simulink model "IMC"  (Simulink 7.6)
settings: Solver=ode45  StartTime=0.0  StopTime=10.0  RelTol=1e-3
values from neighbouring files (symbols this model uses):
  clight = 2.99e8    (= 299000000)    [Generate_IMC_Simulink.m]
  imcl =     [IMC_Filters.mat]
  lambda = 1.064e-6    (= 1.064e-06)    [Generate_IMC_Simulink.m]
  mc2m1l = -1/12*mc2m1l    [ArbLoop_IMC_Simple.m]    (also in IMC_Filters.mat = )
  mc2m2l =     [IMC_Filters.mat]
  mc2m3l = 2.25*mc2m3l    [ArbLoop_IMC_Simple.m]    (also in IMC_Filters.mat = )
  sus =     [sus.mat]
undefined symbols (not defined in the file or in its folder): imc
libraries: cstblocks x42, simulink x16
settings Model: Creator=adammullavey  LastModifiedBy=Chris Mueller
settings DebuggingCC: FcnCallInpInsideContextMsg=Enable All

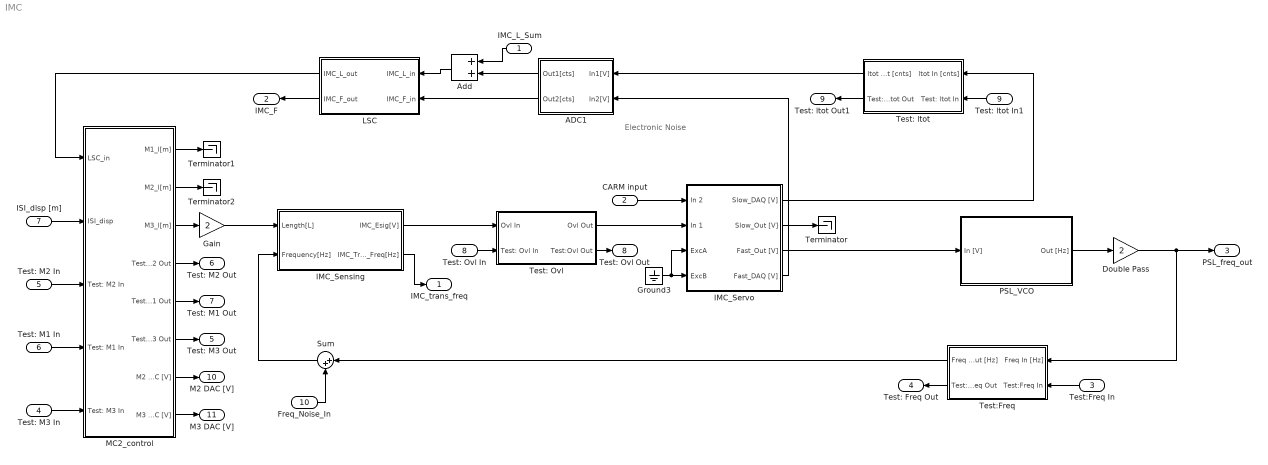
== system IMC ==
  note: Electronic Noise
  IMC_L_Sum : Inport
  CARM input : Inport  Port=2
  Test:Freq In : Inport  Port=3
  Test: M3 In : Inport  Port=4
  Test: M2 In : Inport  Port=5
  Test: M1 In : Inport  Port=6
  ISI_disp [m] : Inport  Port=7
  Test: Ovl In : Inport  Port=8
  Test: ltot In1 : Inport  Port=9
  Freq_Noise_In : Inport  Port=10
  ADC1 : Subsystem
  Add : Sum
  Double Pass : Gain  Gain=2
  Gain : Gain  Gain=2
  Ground3 : Ground
  IMC_Sensing : Subsystem
  IMC_Servo : Subsystem
  LSC : Subsystem
  MC2_control : Subsystem
  PSL_VCO : Subsystem
  Sum : Sum  Inputs=|++
  Terminator : Terminator
  Terminator1 : Terminator
  Terminator2 : Terminator
  Test: Ovl : Subsystem
  Test: ltot : Subsystem
  Test:Freq : Subsystem
  IMC_trans_freq : Outport
  IMC_F : Outport  Port=2
  PSL_freq_out : Outport  Port=3
  Test: Freq Out : Outport  Port=4
  Test: M3 Out : Outport  Port=5
  Test: M2 Out : Outport  Port=6
  Test: M1 Out : Outport  Port=7
  Test: Ovl Out : Outport  Port=8
  Test: ltot Out1 : Outport  Port=9
  M2 DAC [V] : Outport  Port=10
  M3 DAC [V] : Outport  Port=11
  wires:
  Ground3/1 -> IMC_Servo/4(ExcB), IMC_Servo/3(ExcA)
  IMC_Sensing/2(IMC_Trans_Freq[Hz]) -> IMC_trans_freq/1
  IMC_Servo/4(Fast_DAQ [V]) -> ADC1/2(In2[V])
  ADC1/2(Out2[cts]) -> LSC/2(IMC_F_in)
  IMC_Servo/2(Slow_Out [V]) -> Terminator/1
  MC2_control/1(M1_l[m]) -> Terminator1/1
  LSC/2(IMC_F_out) -> IMC_F/1
  PSL_VCO/1(Out [Hz]) -> Double Pass/1
  Double Pass/1 -> PSL_freq_out/1, Test:Freq/1(Freq In [Hz])
  CARM input/1 -> IMC_Servo/1(In 2)
  Gain/1 -> IMC_Sensing/1(Length[L])
  IMC_Servo/3(Fast_Out [V]) -> PSL_VCO/1(In [V])
  Test:Freq In/1 -> Test:Freq/2(Test:Freq In)
  Test:Freq/2(Test:Freq Out) -> Test: Freq Out/1
  LSC/1(IMC_L_out) -> MC2_control/1(LSC_in)
  MC2_control/3(M3_l[m]) -> Gain/1
  MC2_control/2(M2_l[m]) -> Terminator2/1
  Test: M2 In/1 -> MC2_control/3(Test: M2 In)
  MC2_control/4(Test: M2 Out) -> Test: M2 Out/1
  MC2_control/5(Test: M1 Out) -> Test: M1 Out/1
  Test: M1 In/1 -> MC2_control/4(Test: M1 In)
  Test: M3 In/1 -> MC2_control/5(Test: M3 In)
  MC2_control/6(Test: M3 Out) -> Test: M3 Out/1
  Add/1 -> LSC/1(IMC_L_in)
  IMC_L_Sum/1 -> Add/1
  ADC1/1(Out1[cts]) -> Add/2
  ISI_disp [m]/1 -> MC2_control/2(ISI_disp)
  Test: Ovl/2(Test:Ovl Out) -> Test: Ovl Out/1
  Test: Ovl In/1 -> Test: Ovl/2(Test: Ovl In)
  IMC_Sensing/1(IMC_Esig[V]) -> Test: Ovl/1(Ovl In)
  Test: Ovl/1(Ovl Out) -> IMC_Servo/2(In 1)
  Test: ltot/2(Test: ltot Out) -> Test: ltot Out1/1
  Test: ltot In1/1 -> Test: ltot/2(Test: ltot In)
  IMC_Servo/1(Slow_DAQ [V]) -> Test: ltot/1(ltot In [cnts])
  MC2_control/7(M2 DAC [V]) -> M2 DAC [V]/1
  MC2_control/8(M3 DAC [V]) -> M3 DAC [V]/1
  Test: ltot/1(ltot Out [cnts]) -> ADC1/1(In1[V])
  Test:Freq/1(Freq Out [Hz]) -> Sum/1
  Sum/1 -> IMC_Sensing/2(Frequency[Hz])
  Freq_Noise_In/1 -> Sum/2

== system IMC/ADC1 ==
  In1[V] : Inport
  In2[V] : Inport  Port=2
  Gain : Gain  Gain=(2^16)/40
  Gain1 : Gain  Gain=(2^16)/40
  Out1[cts] : Outport
  Out2[cts] : Outport  Port=2
  wires:
  Gain/1 -> Out1[cts]/1
  In1[V]/1 -> Gain/1
  Gain1/1 -> Out2[cts]/1
  In2[V]/1 -> Gain1/1

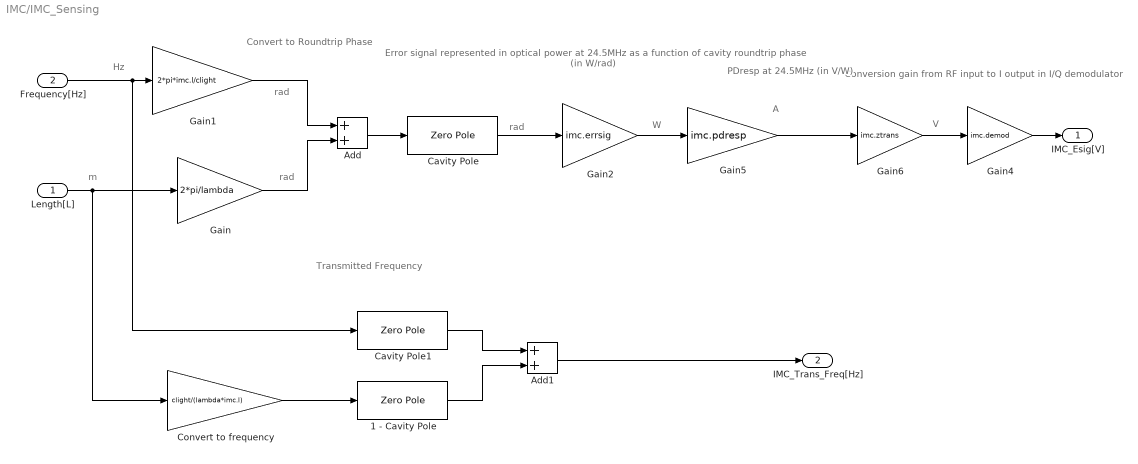
== system IMC/IMC_Sensing ==
  note: Hz
  note: rad
  note: rad
  note: rad
  note: m
  note: V
  note: W
  note: Conversion gain from
      | RF input to I output
      | in I/Q demodulator
  note: Convert to
      | Roundtrip Phase
  note: Error signal represented in
      | optical power at 24.5MHz
      | as a function of cavity
      | roundtrip phase (in W/rad)
  note: Transmitted Frequency
  note: PDresp at 24.5MHz
      |  (in V/W)
  note: A
  Length[L] : Inport
  Frequency[Hz] : Inport  Port=2
  1 - Cavity Pole : ZeroPole  Zeros=[0]  Poles=[-imc.p]  Gain=1
  Add : Sum
  Add1 : Sum
  Cavity Pole : ZeroPole  Zeros=[]  Poles=[-imc.p]  Gain=[imc.p]
  Cavity Pole1 : ZeroPole  Zeros=[]  Poles=[-imc.p]  Gain=[imc.p]
  Convert to frequency : Gain  Gain=clight/(lambda*imc.l)
  Gain : Gain  Gain=2*pi/lambda
  Gain1 : Gain  Gain=2*pi*imc.l/clight
  Gain2 : Gain  Gain=imc.errsig
  Gain4 : Gain  Gain=imc.demod
  Gain5 : Gain  Gain=imc.pdresp
  Gain6 : Gain  Gain=imc.ztrans
  IMC_Esig[V] : Outport
  IMC_Trans_Freq[Hz] : Outport  Port=2
  wires:
  Length[L]/1 -> Convert to frequency/1, Gain/1
  Frequency[Hz]/1 -> Gain1/1, Cavity Pole1/1
  Gain1/1 -> Add/1
  Gain/1 -> Add/2
  Add/1 -> Cavity Pole/1
  Cavity Pole/1 -> Gain2/1
  Add1/1 -> IMC_Trans_Freq[Hz]/1
  Gain4/1 -> IMC_Esig[V]/1
  Gain2/1 -> Gain5/1
  Gain6/1 -> Gain4/1
  Gain5/1 -> Gain6/1
  Cavity Pole1/1 -> Add1/1
  Convert to frequency/1 -> 1 - Cavity Pole/1
  1 - Cavity Pole/1 -> Add1/2

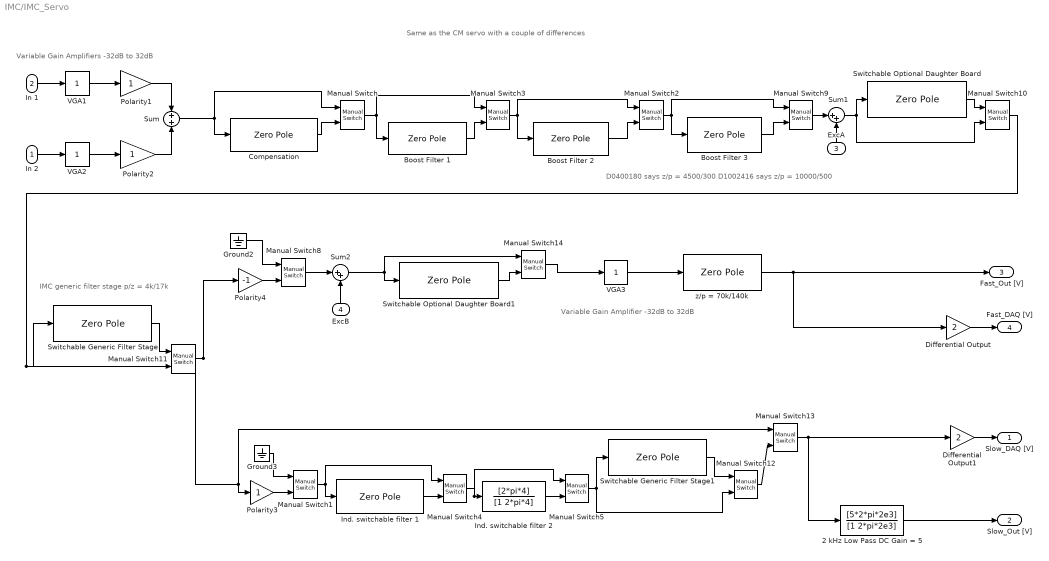
== system IMC/IMC_Servo ==
  note: IMC generic filter stage
      | p/z = 4k/17k
  note: Same as the CM servo with a couple of differences
  note: D0400180 says z/p = 4500/300
      | D1002416 says z/p = 10000/500
  note: Variable Gain Amplifier
      | -32dB to 32dB
  note: Variable Gain Amplifiers
      | -32dB to 32dB
  In 2 : Inport
  In 1 : Inport  Port=2
  ExcA : Inport  Port=3
  ExcB : Inport  Port=4
  2 kHz Low Pass DC Gain = 5 : TransferFcn  Numerator=[5*2*pi*2e3]  Denominator=[1 2*pi*2e3]
  Boost Filter 1 : ZeroPole  Zeros=-2*pi*[20e3]  Poles=-2*pi*[1e3]
  Boost Filter 2 : ZeroPole  Zeros=-2*pi*[20e3]  Poles=-2*pi*[1e3]
  Boost Filter 3 : ZeroPole  Zeros=-2*pi*[10e3]  Poles=-2*pi*[500]
  Compensation : ZeroPole  Zeros=-2*pi*[4e3]  Poles=-2*pi*[40]
  Differential Output : Gain  Gain=2
  Differential Output1 : Gain  Gain=2
  Ground2 : Ground
  Ground3 : Ground
  Ind. switchable filter 1 : ZeroPole  Zeros=-2*pi*[400]  Poles=-2*pi*[4]  Gain=[1/100]
  Ind. switchable filter 2 : TransferFcn  Numerator=[2*pi*4]  Denominator=[1 2*pi*4]
  Manual Switch{,1,3..4,8,10..12} (8 alike) : simulink/Signal Routing/Manual Switch  SystemSampleTime=-1  sw=0  action=0  varsize=off
  Manual Switch{2,5,9,13..14} (5 alike) : simulink/Signal Routing/Manual Switch  SystemSampleTime=-1  sw=1  action=0  varsize=off
  Polarity1 : Gain
  Polarity2 : Gain
  Polarity3 : Gain
  Polarity4 : Gain  Gain=-1
  Sum : Sum  Inputs=+|+
  Sum1 : Sum  Inputs=|++
  Sum2 : Sum  Inputs=|++
  Switchable Generic Filter Stage : ZeroPole  Zeros=-2*pi*[17e3]  Poles=-2*pi*[4e3]  Gain=[4/17]
  Switchable Generic Filter Stage1 : ZeroPole  Zeros=-2*pi*[500]  Poles=-2*pi*[1e4]  Gain=[1e4/500]
  Switchable Optional Daughter Board : ZeroPole  Zeros=-2*pi*[500]  Poles=-2*pi*[1e4]  Gain=[1e4/500]
  Switchable Optional Daughter Board1 : ZeroPole  Zeros=-2*pi*[500]  Poles=-2*pi*[1e4]  Gain=[1e4/500]
  VGA1 : simulink/Math Operations/Slider Gain  SystemSampleTime=-1  low=0.025  gain=1  high=40
  VGA2 : simulink/Math Operations/Slider Gain  SystemSampleTime=-1  low=0.025  gain=1  high=40
  VGA3 : simulink/Math Operations/Slider Gain  SystemSampleTime=-1  low=0.025  gain=1  high=40
  z/p = 70k/140k : ZeroPole  Zeros=-2*pi*[70000]  Poles=-2*pi*[140000]  Gain=2
  Slow_DAQ [V] : Outport
  Slow_Out [V] : Outport  Port=2
  Fast_Out [V] : Outport  Port=3
  Fast_DAQ [V] : Outport  Port=4
  wires:
  Polarity1/1 -> Sum/1
  VGA1/1 -> Polarity1/1
  In 1/1 -> VGA1/1
  VGA3/1 -> z/p = 70k/140k/1
  VGA2/1 -> Polarity2/1
  In 2/1 -> VGA2/1
  Switchable Generic Filter Stage1/1 -> Manual Switch12/1
  Ground3/1 -> Manual Switch1/1
  Ground2/1 -> Manual Switch8/1
  Switchable Optional Daughter Board1/1 -> Manual Switch14/2
  Compensation/1 -> Manual Switch/2
  Manual Switch/1 -> Manual Switch3/1, Boost Filter 1/1
  Boost Filter 1/1 -> Manual Switch3/2
  Manual Switch3/1 -> Manual Switch2/1, Boost Filter 2/1
  Boost Filter 2/1 -> Manual Switch2/2
  Switchable Optional Daughter Board/1 -> Manual Switch10/1
  Manual Switch1/1 -> Manual Switch4/1, Ind. switchable filter 1/1
  Manual Switch4/1 -> Manual Switch5/1, Ind. switchable filter 2/1
  Manual Switch5/1 -> Switchable Generic Filter Stage1/1, Manual Switch12/2
  Ind. switchable filter 2/1 -> Manual Switch5/2
  Sum/1 -> Manual Switch/1, Compensation/1
  ExcB/1 -> Sum2/2
  Manual Switch8/1 -> Sum2/1
  z/p = 70k/140k/1 -> Fast_Out [V]/1, Differential Output/1
  Polarity2/1 -> Sum/2
  ExcA/1 -> Sum1/2
  Boost Filter 3/1 -> Manual Switch9/2
  Manual Switch9/1 -> Sum1/1
  Manual Switch2/1 -> Manual Switch9/1, Boost Filter 3/1
  Ind. switchable filter 1/1 -> Manual Switch4/2
  Sum1/1 -> Switchable Optional Daughter Board/1, Manual Switch10/2
  Manual Switch10/1 -> Switchable Generic Filter Stage/1, Manual Switch11/2
  Switchable Generic Filter Stage/1 -> Manual Switch11/1
  Manual Switch11/1 -> Manual Switch13/1, Polarity3/1, Polarity4/1
  Manual Switch12/1 -> Manual Switch13/2
  Sum2/1 -> Switchable Optional Daughter Board1/1, Manual Switch14/1
  Manual Switch14/1 -> VGA3/1
  Polarity4/1 -> Manual Switch8/2
  Polarity3/1 -> Manual Switch1/2
  Manual Switch13/1 -> 2 kHz Low Pass DC Gain = 5/1, Differential Output1/1
  Differential Output/1 -> Fast_DAQ [V]/1
  2 kHz Low Pass DC Gain = 5/1 -> Slow_Out [V]/1
  Differential Output1/1 -> Slow_DAQ [V]/1

== system IMC/LSC ==
  note: Copied from foton
  IMC_L_in : Inport
  IMC_F_in : Inport  Port=2
  IMC-L Filter Bank : Subsystem
  InvGenFilt : ZeroPole  Zeros=-2*pi*[100 100]  Poles=-2*pi*[10 10]  Gain=[0.01/2]
  VCO  filter [cts/cts]:  pole:1.6 Hz; zero:40 Hz : ZeroPole  Zeros=-2*pi*[40]  Poles=-2*pi*[1.6]  Gain=1.4906e6*(1.6/40)
  ctstoV : Gain  Gain=6.10016e-4
  IMC_L_out : Outport
  IMC_F_out : Outport  Port=2
  wires:
  IMC_L_in/1 -> IMC-L Filter Bank/1(In1)
  IMC-L Filter Bank/1(Out1) -> IMC_L_out/1
  IMC_F_in/1 -> InvGenFilt/1
  InvGenFilt/1 -> VCO  filter [cts/cts]:  pole:1.6 Hz; zero:40 Hz/1
  VCO  filter [cts/cts]:  pole:1.6 Hz; zero:40 Hz/1 -> ctstoV/1
  ctstoV/1 -> IMC_F_out/1

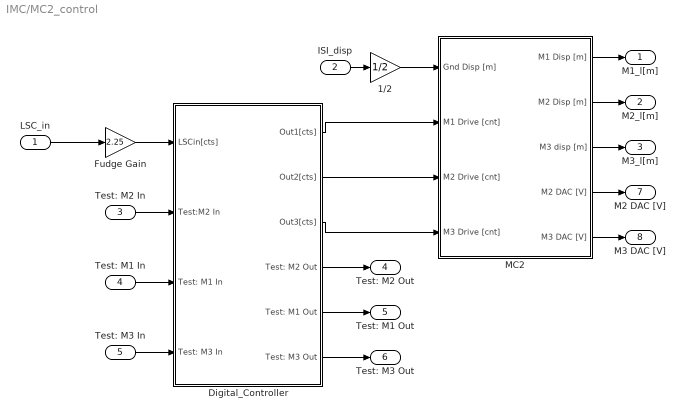
== system IMC/MC2_control ==
  LSC_in : Inport
  ISI_disp : Inport  Port=2
  Test: M2 In : Inport  Port=3
  Test: M1 In : Inport  Port=4
  Test: M3 In : Inport  Port=5
  1/2 : Gain  Gain=1/2
  Digital_Controller : Subsystem
  Fudge Gain : Gain  Gain=2.25
  MC2 : Subsystem
  M1_l[m] : Outport
  M2_l[m] : Outport  Port=2
  M3_l[m] : Outport  Port=3
  Test: M2 Out : Outport  Port=4
  Test: M1 Out : Outport  Port=5
  Test: M3 Out : Outport  Port=6
  M2 DAC [V] : Outport  Port=7
  M3 DAC [V] : Outport  Port=8
  wires:
  ISI_disp/1 -> 1/2/1
  MC2/2(M2 Disp [m]) -> M2_l[m]/1
  MC2/1(M1 Disp [m]) -> M1_l[m]/1
  MC2/3(M3 disp [m]) -> M3_l[m]/1
  Digital_Controller/1(Out1[cts]) -> MC2/2(M1 Drive [cnt])
  Digital_Controller/2(Out2[cts]) -> MC2/3(M2 Drive [cnt])
  Digital_Controller/3(Out3[cts]) -> MC2/4(M3 Drive [cnt])
  LSC_in/1 -> Fudge Gain/1
  Test: M2 In/1 -> Digital_Controller/2(Test:M2 In)
  Test: M1 In/1 -> Digital_Controller/3(Test: M1 In)
  Digital_Controller/4(Test: M2 Out) -> Test: M2 Out/1
  Digital_Controller/5(Test: M1 Out) -> Test: M1 Out/1
  Test: M3 In/1 -> Digital_Controller/4(Test: M3 In)
  Digital_Controller/6(Test: M3 Out) -> Test: M3 Out/1
  Fudge Gain/1 -> Digital_Controller/1(LSCin[cts])
  MC2/4(M2 DAC [V]) -> M2 DAC [V]/1
  MC2/5(M3 DAC [V]) -> M3 DAC [V]/1
  1/2/1 -> MC2/1(Gnd Disp [m])

== system IMC/PSL_VCO ==
  note: Output range of +/-1MHz (79-81MHz), Input range +/-20V, hence sensitivity 1MHz/20V. Just an approximation, really should be measured.
  note: Low Noise VCO - described in T0900451, schematics in D0900605-A
  note: P/Z = 275kHz/2750kHz
  note: 1MHz/20V
  note: llo alog 4090 - old VCO = 745300Hz/V
  note: valera says new vco = old vco/3
      | therefore new vco = 2.4843e5 Hz/V
  In [V] : Inport
  VCO  filter [V/V]:  pole:1.6 Hz; zero:40 Hz : ZeroPole  Zeros=-2*pi*[40]  Poles=-2*pi*[1.6]  Gain=(1.6/40)
  VCO TF req - 20 deg phase shift at 50 kHz : ZeroPole  Zeros=-2*pi*[2750e3]  Poles=-2*pi*[275e3]  Gain=(1/10)
  VCO gain [Hz/V] : Gain  Gain=2.4843e5  SaturateOnIntegerOverflow=on  OutDataTypeStr=Inherit: Same as input  ParamDataTypeStr=Inherit: Same as input
  Out [Hz] : Outport
  wires:
  In [V]/1 -> VCO  filter [V/V]:  pole:1.6 Hz; zero:40 Hz/1
  VCO gain [Hz/V]/1 -> Out [Hz]/1
  VCO  filter [V/V]:  pole:1.6 Hz; zero:40 Hz/1 -> VCO TF req - 20 deg phase shift at 50 kHz/1
  VCO TF req - 20 deg phase shift at 50 kHz/1 -> VCO gain [Hz/V]/1

== system IMC/Test: Ovl ==
  Ovl In : Inport
  Test: Ovl In : Inport  Port=2
  Add : Sum
  Constant : Constant  Value=imc.sw.ovl
  Ground : Ground
  Switch : Switch  Threshold=0.5
  Ovl Out : Outport
  Test:Ovl Out : Outport  Port=2
  wires:
  Ground/1 -> Switch/3
  Constant/1 -> Switch/2
  Ovl In/1 -> Switch/1, Test:Ovl Out/1
  Switch/1 -> Add/2
  Test: Ovl In/1 -> Add/1
  Add/1 -> Ovl Out/1

== system IMC/Test: ltot ==
  ltot In [cnts] : Inport
  Test: ltot In : Inport  Port=2
  Add : Sum
  Constant : Constant  Value=imc.sw.ltot
  Ground : Ground
  Switch : Switch  Threshold=0.5
  ltot Out [cnts] : Outport
  Test: ltot Out : Outport  Port=2
  wires:
  Add/1 -> ltot Out [cnts]/1
  Test: ltot In/1 -> Add/1
  Switch/1 -> Add/2
  ltot In [cnts]/1 -> Test: ltot Out/1, Switch/1
  Constant/1 -> Switch/2
  Ground/1 -> Switch/3

== system IMC/Test:Freq ==
  Freq In [Hz] : Inport
  Test:Freq In : Inport  Port=2
  Add : Sum
  Constant : Constant  Value=imc.sw.freq
  Ground : Ground
  Switch : Switch  Threshold=0.5
  Freq Out [Hz] : Outport
  Test:Freq Out : Outport  Port=2
  wires:
  Ground/1 -> Switch/3
  Constant/1 -> Switch/2
  Freq In [Hz]/1 -> Switch/1, Test:Freq Out/1
  Switch/1 -> Add/2
  Test:Freq In/1 -> Add/1
  Add/1 -> Freq Out [Hz]/1

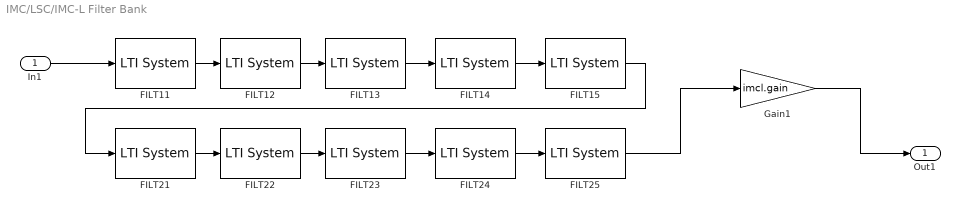
== system IMC/LSC/IMC-L Filter Bank ==
  In1 : Inport
  FILT11 : cstblocks/LTI System  SystemSampleTime=-1  sys=imcl.filts(1).sys  IC=[]
  FILT12 : cstblocks/LTI System  SystemSampleTime=-1  sys=imcl.filts(2).sys  IC=[]
  FILT13 : cstblocks/LTI System  SystemSampleTime=-1  sys=imcl.filts(3).sys  IC=[]
  FILT14 : cstblocks/LTI System  SystemSampleTime=-1  sys=imcl.filts(4).sys  IC=[]
  FILT15 : cstblocks/LTI System  SystemSampleTime=-1  sys=imcl.filts(5).sys  IC=[]
  FILT21 : cstblocks/LTI System  SystemSampleTime=-1  sys=imcl.filts(6).sys  IC=[]
  FILT22 : cstblocks/LTI System  SystemSampleTime=-1  sys=imcl.filts(7).sys  IC=[]
  FILT23 : cstblocks/LTI System  SystemSampleTime=-1  sys=imcl.filts(8).sys  IC=[]
  FILT24 : cstblocks/LTI System  SystemSampleTime=-1  sys=imcl.filts(9).sys  IC=[]
  FILT25 : cstblocks/LTI System  SystemSampleTime=-1  sys=imcl.filts(10).sys  IC=[]
  Gain1 : Gain  Gain=imcl.gain
  Out1 : Outport
  wires:
  FILT11/1 -> FILT12/1
  FILT12/1 -> FILT13/1
  FILT13/1 -> FILT14/1
  FILT14/1 -> FILT15/1
  FILT21/1 -> FILT22/1
  FILT22/1 -> FILT23/1
  FILT23/1 -> FILT24/1
  FILT24/1 -> FILT25/1
  In1/1 -> FILT11/1
  FILT15/1 -> FILT21/1
  FILT25/1 -> Gain1/1
  Gain1/1 -> Out1/1

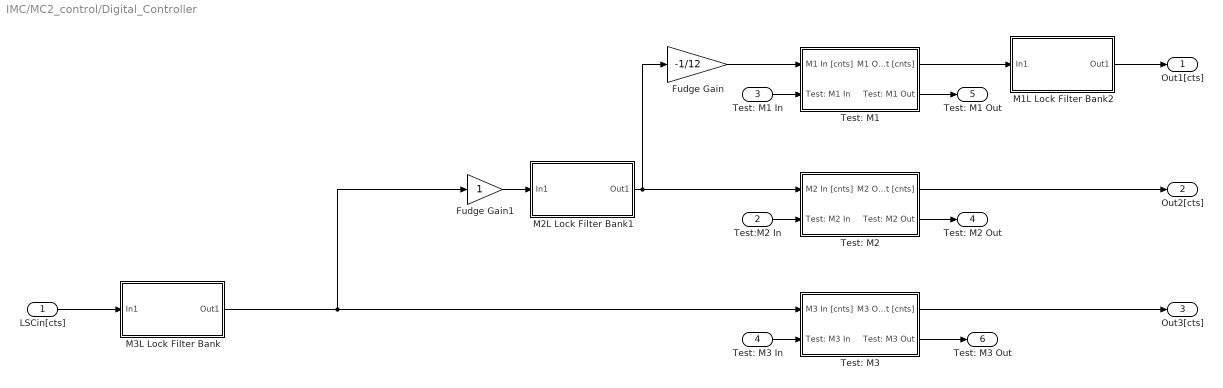
== system IMC/MC2_control/Digital_Controller ==
  LSCin[cts] : Inport
  Test:M2 In : Inport  Port=2
  Test: M1 In : Inport  Port=3
  Test: M3 In : Inport  Port=4
  Fudge Gain : Gain  Gain=-1/12
  Fudge Gain1 : Gain
  M1L Lock Filter Bank2 : Subsystem
  M2L Lock Filter Bank1 : Subsystem
  M3L Lock Filter Bank : Subsystem
  Test: M1 : Subsystem
  Test: M2 : Subsystem
  Test: M3 : Subsystem
  Out1[cts] : Outport
  Out2[cts] : Outport  Port=2
  Out3[cts] : Outport  Port=3
  Test: M2 Out : Outport  Port=4
  Test: M1 Out : Outport  Port=5
  Test: M3 Out : Outport  Port=6
  wires:
  M2L Lock Filter Bank1/1(Out1) -> Test: M2/1(M2 In [cnts]), Fudge Gain/1
  LSCin[cts]/1 -> M3L Lock Filter Bank/1(In1)
  M1L Lock Filter Bank2/1(Out1) -> Out1[cts]/1
  Test:M2 In/1 -> Test: M2/2(Test: M2 In)
  Test: M2/2(Test: M2 Out) -> Test: M2 Out/1
  Test: M1 In/1 -> Test: M1/2(Test: M1 In)
  Test: M1/2(Test: M1 Out) -> Test: M1 Out/1
  Test: M1/1(M1 Out [cnts]) -> M1L Lock Filter Bank2/1(In1)
  Test: M2/1(M2 Out [cnts]) -> Out2[cts]/1
  Test: M3/2(Test: M3 Out) -> Test: M3 Out/1
  Test: M3 In/1 -> Test: M3/2(Test: M3 In)
  Test: M3/1(M3 Out [cnts]) -> Out3[cts]/1
  Fudge Gain1/1 -> M2L Lock Filter Bank1/1(In1)
  M3L Lock Filter Bank/1(Out1) -> Fudge Gain1/1, Test: M3/1(M3 In [cnts])
  Fudge Gain/1 -> Test: M1/1(M1 In [cnts])

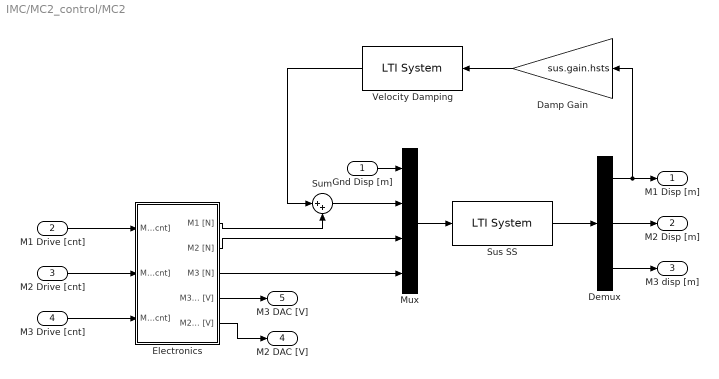
== system IMC/MC2_control/MC2 ==
  Gnd Disp [m] : Inport
  M1 Drive [cnt] : Inport  Port=2
  M2 Drive [cnt] : Inport  Port=3
  M3 Drive [cnt] : Inport  Port=4
  Damp Gain : Gain  Gain=sus.gain.hsts
  Demux : Demux  Outputs=3
  Electronics : Subsystem
  Mux : Mux
  Sum : Sum  Inputs=|++
  Sus SS : cstblocks/LTI System  SystemSampleTime=-1  sys=sus.hsts.ss  IC=[]
  Velocity Damping : cstblocks/LTI System  SystemSampleTime=-1  sys=sus.damp  IC=[]
  M1 Disp [m] : Outport
  M2 Disp [m] : Outport  Port=2
  M3 disp [m] : Outport  Port=3
  M2 DAC [V] : Outport  Port=4
  M3 DAC [V] : Outport  Port=5
  wires:
  Mux/1 -> Sus SS/1
  Gnd Disp [m]/1 -> Mux/1
  Sus SS/1 -> Demux/1
  Demux/3 -> M3 disp [m]/1
  Demux/2 -> M2 Disp [m]/1
  Demux/1 -> M1 Disp [m]/1, Damp Gain/1
  Sum/1 -> Mux/2
  Velocity Damping/1 -> Sum/1
  Damp Gain/1 -> Velocity Damping/1
  Electronics/1(M1 [N]) -> Sum/2
  Electronics/2(M2 [N]) -> Mux/3
  Electronics/3(M3 [N]) -> Mux/4
  M1 Drive [cnt]/1 -> Electronics/1(M1 [cnt])
  M2 Drive [cnt]/1 -> Electronics/2(M2 [cnt])
  M3 Drive [cnt]/1 -> Electronics/3(M3 [cnt])
  Electronics/5(M2 DAC [V]) -> M2 DAC [V]/1
  Electronics/4(M3 DAC [V]) -> M3 DAC [V]/1

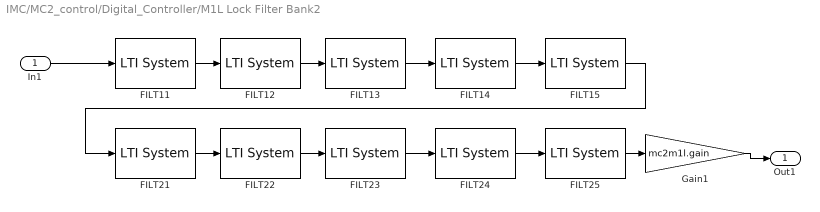
== system IMC/MC2_control/Digital_Controller/M1L Lock Filter Bank2 ==
  In1 : Inport
  FILT11 : cstblocks/LTI System  SystemSampleTime=-1  sys=mc2m1l.filts(1).sys  IC=[]
  FILT12 : cstblocks/LTI System  SystemSampleTime=-1  sys=mc2m1l.filts(2).sys  IC=[]
  FILT13 : cstblocks/LTI System  SystemSampleTime=-1  sys=mc2m1l.filts(3).sys  IC=[]
  FILT14 : cstblocks/LTI System  SystemSampleTime=-1  sys=mc2m1l.filts(4).sys  IC=[]
  FILT15 : cstblocks/LTI System  SystemSampleTime=-1  sys=mc2m1l.filts(5).sys  IC=[]
  FILT21 : cstblocks/LTI System  SystemSampleTime=-1  sys=mc2m1l.filts(6).sys  IC=[]
  FILT22 : cstblocks/LTI System  SystemSampleTime=-1  sys=mc2m1l.filts(7).sys  IC=[]
  FILT23 : cstblocks/LTI System  SystemSampleTime=-1  sys=mc2m1l.filts(8).sys  IC=[]
  FILT24 : cstblocks/LTI System  SystemSampleTime=-1  sys=mc2m1l.filts(9).sys  IC=[]
  FILT25 : cstblocks/LTI System  SystemSampleTime=-1  sys=mc2m1l.filts(10).sys  IC=[]
  Gain1 : Gain  Gain=mc2m1l.gain
  Out1 : Outport
  wires:
  FILT15/1 -> FILT21/1
  Gain1/1 -> Out1/1
  In1/1 -> FILT11/1
  FILT25/1 -> Gain1/1
  FILT24/1 -> FILT25/1
  FILT23/1 -> FILT24/1
  FILT22/1 -> FILT23/1
  FILT21/1 -> FILT22/1
  FILT14/1 -> FILT15/1
  FILT13/1 -> FILT14/1
  FILT12/1 -> FILT13/1
  FILT11/1 -> FILT12/1

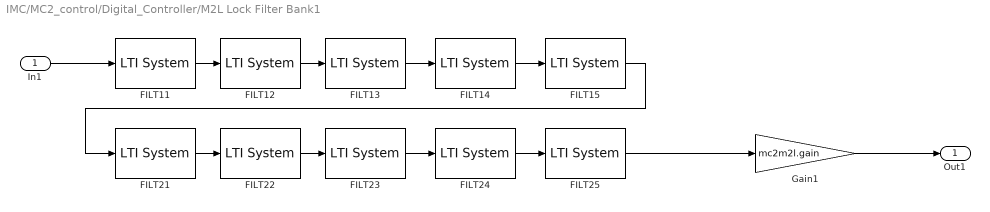
== system IMC/MC2_control/Digital_Controller/M2L Lock Filter Bank1 ==
  In1 : Inport
  FILT11 : cstblocks/LTI System  SystemSampleTime=-1  sys=mc2m2l.filts(1).sys  IC=[]
  FILT12 : cstblocks/LTI System  SystemSampleTime=-1  sys=mc2m2l.filts(2).sys  IC=[]
  FILT13 : cstblocks/LTI System  SystemSampleTime=-1  sys=mc2m2l.filts(3).sys  IC=[]
  FILT14 : cstblocks/LTI System  SystemSampleTime=-1  sys=mc2m2l.filts(4).sys  IC=[]
  FILT15 : cstblocks/LTI System  SystemSampleTime=-1  sys=mc2m2l.filts(5).sys  IC=[]
  FILT21 : cstblocks/LTI System  SystemSampleTime=-1  sys=mc2m2l.filts(6).sys  IC=[]
  FILT22 : cstblocks/LTI System  SystemSampleTime=-1  sys=mc2m2l.filts(7).sys  IC=[]
  FILT23 : cstblocks/LTI System  SystemSampleTime=-1  sys=mc2m2l.filts(8).sys  IC=[]
  FILT24 : cstblocks/LTI System  SystemSampleTime=-1  sys=mc2m2l.filts(9).sys  IC=[]
  FILT25 : cstblocks/LTI System  SystemSampleTime=-1  sys=mc2m2l.filts(10).sys  IC=[]
  Gain1 : Gain  Gain=mc2m2l.gain
  Out1 : Outport
  wires:
  FILT11/1 -> FILT12/1
  FILT12/1 -> FILT13/1
  FILT13/1 -> FILT14/1
  FILT14/1 -> FILT15/1
  FILT21/1 -> FILT22/1
  FILT22/1 -> FILT23/1
  FILT23/1 -> FILT24/1
  FILT24/1 -> FILT25/1
  In1/1 -> FILT11/1
  FILT15/1 -> FILT21/1
  Gain1/1 -> Out1/1
  FILT25/1 -> Gain1/1

== system IMC/MC2_control/Digital_Controller/M3L Lock Filter Bank ==
  In1 : Inport
  FILT11 : cstblocks/LTI System  SystemSampleTime=-1  sys=mc2m3l.filts(1).sys  IC=[]
  FILT12 : cstblocks/LTI System  SystemSampleTime=-1  sys=mc2m3l.filts(2).sys  IC=[]
  FILT13 : cstblocks/LTI System  SystemSampleTime=-1  sys=mc2m3l.filts(3).sys  IC=[]
  FILT14 : cstblocks/LTI System  SystemSampleTime=-1  sys=mc2m3l.filts(4).sys  IC=[]
  FILT15 : cstblocks/LTI System  SystemSampleTime=-1  sys=mc2m3l.filts(5).sys  IC=[]
  FILT21 : cstblocks/LTI System  SystemSampleTime=-1  sys=mc2m3l.filts(6).sys  IC=[]
  FILT22 : cstblocks/LTI System  SystemSampleTime=-1  sys=mc2m3l.filts(7).sys  IC=[]
  FILT23 : cstblocks/LTI System  SystemSampleTime=-1  sys=mc2m3l.filts(8).sys  IC=[]
  FILT24 : cstblocks/LTI System  SystemSampleTime=-1  sys=mc2m3l.filts(9).sys  IC=[]
  FILT25 : cstblocks/LTI System  SystemSampleTime=-1  sys=mc2m3l.filts(10).sys  IC=[]
  Gain1 : Gain  Gain=mc2m3l.gain
  Out1 : Outport
  wires:
  FILT15/1 -> FILT21/1
  Gain1/1 -> Out1/1
  In1/1 -> FILT11/1
  FILT25/1 -> Gain1/1
  FILT24/1 -> FILT25/1
  FILT23/1 -> FILT24/1
  FILT22/1 -> FILT23/1
  FILT21/1 -> FILT22/1
  FILT14/1 -> FILT15/1
  FILT13/1 -> FILT14/1
  FILT12/1 -> FILT13/1
  FILT11/1 -> FILT12/1

== system IMC/MC2_control/Digital_Controller/Test: M1 ==
  M1 In [cnts] : Inport
  Test: M1 In : Inport  Port=2
  Add : Sum
  Constant : Constant  Value=imc.sw.m1
  Ground : Ground
  Switch : Switch  Threshold=0.5
  M1 Out [cnts] : Outport
  Test: M1 Out : Outport  Port=2
  wires:
  Ground/1 -> Switch/3
  Constant/1 -> Switch/2
  M1 In [cnts]/1 -> Switch/1, Test: M1 Out/1
  Switch/1 -> Add/2
  Test: M1 In/1 -> Add/1
  Add/1 -> M1 Out [cnts]/1

== system IMC/MC2_control/Digital_Controller/Test: M2 ==
  M2 In [cnts] : Inport
  Test: M2 In : Inport  Port=2
  Add : Sum
  Constant : Constant  Value=imc.sw.m2
  Ground : Ground
  Switch : Switch  Threshold=0.5
  M2 Out [cnts] : Outport
  Test: M2 Out : Outport  Port=2
  wires:
  Ground/1 -> Switch/3
  Constant/1 -> Switch/2
  M2 In [cnts]/1 -> Switch/1, Test: M2 Out/1
  Switch/1 -> Add/2
  Test: M2 In/1 -> Add/1
  Add/1 -> M2 Out [cnts]/1

== system IMC/MC2_control/Digital_Controller/Test: M3 ==
  M3 In [cnts] : Inport
  Test: M3 In : Inport  Port=2
  Add : Sum
  Constant : Constant  Value=imc.sw.m3
  Ground : Ground
  Switch : Switch  Threshold=0.5
  M3 Out [cnts] : Outport
  Test: M3 Out : Outport  Port=2
  wires:
  Add/1 -> M3 Out [cnts]/1
  Test: M3 In/1 -> Add/1
  Switch/1 -> Add/2
  M3 In [cnts]/1 -> Test: M3 Out/1, Switch/1
  Constant/1 -> Switch/2
  Ground/1 -> Switch/3

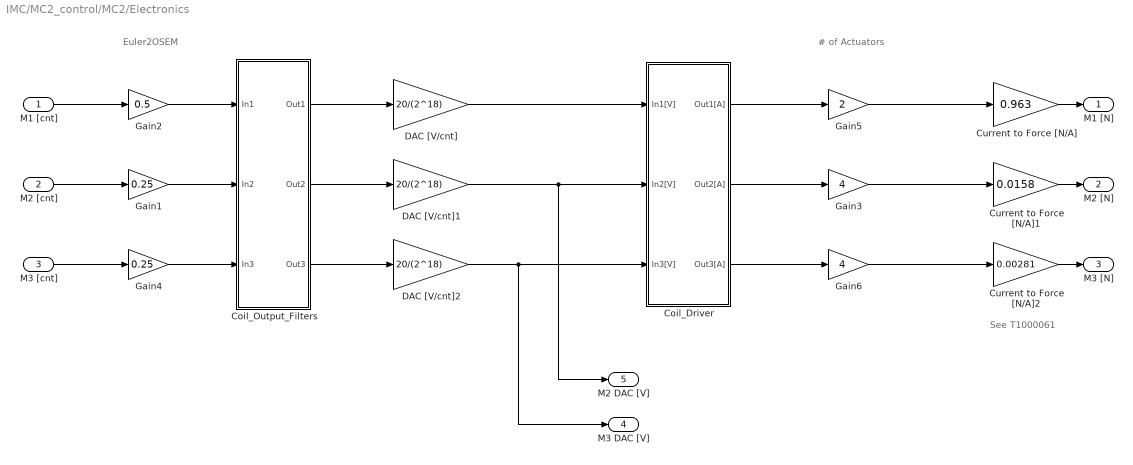
== system IMC/MC2_control/MC2/Electronics ==
  note: See T1000061
  note: Euler2OSEM
  note: # of Actuators
  M1 [cnt] : Inport
  M2 [cnt] : Inport  Port=2
  M3 [cnt] : Inport  Port=3
  Coil_Driver : Subsystem
  Coil_Output_Filters : Subsystem
  Current to Force [N/A] : Gain  Gain=0.963
  Current to Force [N/A]1 : Gain  Gain=0.0158
  Current to Force [N/A]2 : Gain  Gain=0.00281
  DAC [V/cnt] : Gain  Gain=20/(2^18)
  DAC [V/cnt]1 : Gain  Gain=20/(2^18)
  DAC [V/cnt]2 : Gain  Gain=20/(2^18)
  Gain1 : Gain  Gain=0.25
  Gain2 : Gain  Gain=0.5
  Gain3 : Gain  Gain=4
  Gain4 : Gain  Gain=0.25
  Gain5 : Gain  Gain=2
  Gain6 : Gain  Gain=4
  M1 [N] : Outport
  M2 [N] : Outport  Port=2
  M3 [N] : Outport  Port=3
  M3 DAC [V] : Outport  Port=4
  M2 DAC [V] : Outport  Port=5
  wires:
  Current to Force [N/A]/1 -> M1 [N]/1
  Current to Force [N/A]1/1 -> M2 [N]/1
  Current to Force [N/A]2/1 -> M3 [N]/1
  DAC [V/cnt]1/1 -> M2 DAC [V]/1, Coil_Driver/2(In2[V])
  DAC [V/cnt]2/1 -> M3 DAC [V]/1, Coil_Driver/3(In3[V])
  Gain2/1 -> Coil_Output_Filters/1(In1)
  Gain1/1 -> Coil_Output_Filters/2(In2)
  Gain4/1 -> Coil_Output_Filters/3(In3)
  Coil_Output_Filters/1(Out1) -> DAC [V/cnt]/1
  Coil_Output_Filters/2(Out2) -> DAC [V/cnt]1/1
  Coil_Output_Filters/3(Out3) -> DAC [V/cnt]2/1
  M1 [cnt]/1 -> Gain2/1
  M2 [cnt]/1 -> Gain1/1
  M3 [cnt]/1 -> Gain4/1
  DAC [V/cnt]/1 -> Coil_Driver/1(In1[V])
  Gain5/1 -> Current to Force [N/A]/1
  Gain3/1 -> Current to Force [N/A]1/1
  Gain6/1 -> Current to Force [N/A]2/1
  Coil_Driver/1(Out1[A]) -> Gain5/1
  Coil_Driver/2(Out2[A]) -> Gain3/1
  Coil_Driver/3(Out3[A]) -> Gain6/1

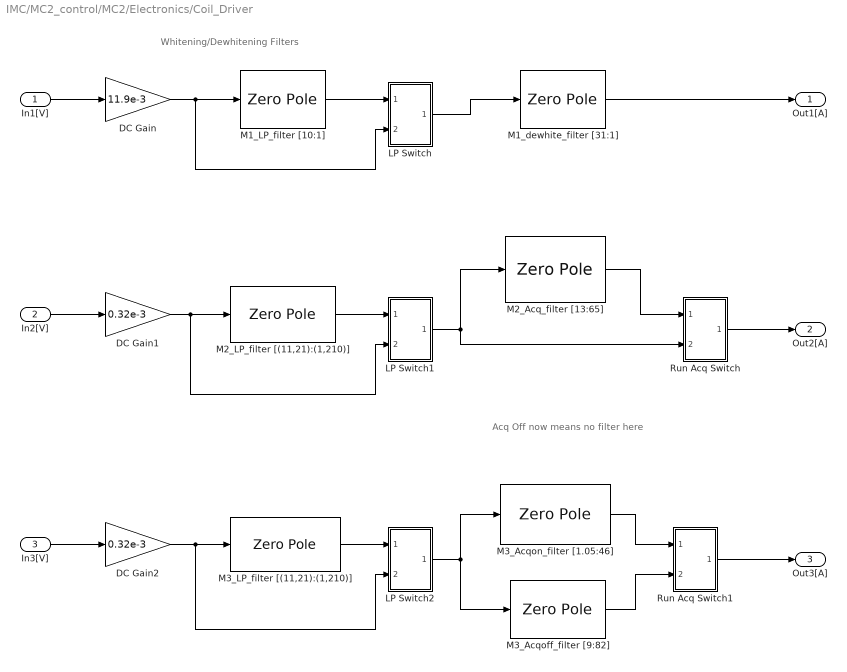
== system IMC/MC2_control/MC2/Electronics/Coil_Driver ==
  note: Whitening/Dewhitening Filters
  note: Acq Off now means no filter here
  In1[V] : Inport
  In2[V] : Inport  Port=2
  In3[V] : Inport  Port=3
  DC Gain : Gain  Gain=11.9e-3
  DC Gain1 : Gain  Gain=0.32e-3
  DC Gain2 : Gain  Gain=0.32e-3
  LP Switch : Subsystem
  LP Switch1 : Subsystem
  LP Switch2 : Subsystem
  M1_LP_filter [10:1] : ZeroPole  Zeros=-2*pi*[10]  Poles=-2*pi*[1]  Gain=[1/10]
  M1_dewhite_filter [31:1] : ZeroPole  Zeros=-2*pi*[31]  Poles=-2*pi*[1]  Gain=[1/31]
  M2_Acq_filter [13:65] : ZeroPole  Zeros=-2*pi*[13]  Poles=-2*pi*[65]  Gain=[65/13]
  M2_LP_filter [(11,21):(1,210)] : ZeroPole  Zeros=-2*pi*[11 21]  Poles=-2*pi*[1 210]  Gain=[10/11]
  M3_Acqoff_filter [9:82] : ZeroPole  Zeros=-2*pi*[9]  Poles=-2*pi*[82]  Gain=[82/9]
  M3_Acqon_filter [1.05:46] : ZeroPole  Zeros=-2*pi*[1.05]  Poles=-2*pi*[46]  Gain=[46/1.05]
  M3_LP_filter [(11,21):(1,210)] : ZeroPole  Zeros=-2*pi*[11 21]  Poles=-2*pi*[1 210]  Gain=[10/11]
  Run Acq Switch : Subsystem
  Run Acq Switch1 : Subsystem
  Out1[A] : Outport
  Out2[A] : Outport  Port=2
  Out3[A] : Outport  Port=3
  wires:
  In1[V]/1 -> DC Gain/1
  DC Gain/1 -> M1_LP_filter [10:1]/1, LP Switch/2(In5)
  In3[V]/1 -> DC Gain2/1
  DC Gain2/1 -> M3_LP_filter [(11,21):(1,210)]/1, LP Switch2/2(In5)
  In2[V]/1 -> DC Gain1/1
  DC Gain1/1 -> M2_LP_filter [(11,21):(1,210)]/1, LP Switch1/2(In5)
  M1_dewhite_filter [31:1]/1 -> Out1[A]/1
  M3_LP_filter [(11,21):(1,210)]/1 -> LP Switch2/1(In4)
  M2_LP_filter [(11,21):(1,210)]/1 -> LP Switch1/1(In4)
  M1_LP_filter [10:1]/1 -> LP Switch/1(In4)
  LP Switch/1(Out4) -> M1_dewhite_filter [31:1]/1
  LP Switch1/1(Out4) -> M2_Acq_filter [13:65]/1, Run Acq Switch/2(In5)
  LP Switch2/1(Out4) -> M3_Acqon_filter [1.05:46]/1, M3_Acqoff_filter [9:82]/1
  Run Acq Switch/1(Out4) -> Out2[A]/1
  M2_Acq_filter [13:65]/1 -> Run Acq Switch/1(In4)
  Run Acq Switch1/1(Out4) -> Out3[A]/1
  M3_Acqon_filter [1.05:46]/1 -> Run Acq Switch1/1(In4)
  M3_Acqoff_filter [9:82]/1 -> Run Acq Switch1/2(In5)

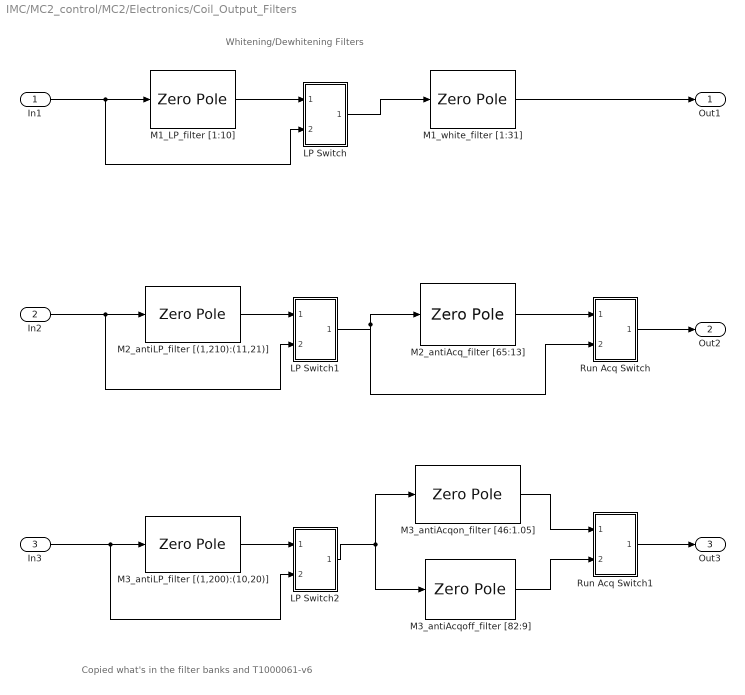
== system IMC/MC2_control/MC2/Electronics/Coil_Output_Filters ==
  note: Whitening/Dewhitening Filters
  note: Copied what's in the filter banks and T1000061-v6
  In1 : Inport
  In2 : Inport  Port=2
  In3 : Inport  Port=3
  LP Switch : Subsystem
  LP Switch1 : Subsystem
  LP Switch2 : Subsystem
  M1_LP_filter [1:10] : ZeroPole  Zeros=-2*pi*[1]  Poles=-2*pi*[10]  Gain=[10/1]
  M1_white_filter [1:31] : ZeroPole  Zeros=-2*pi*[1]  Poles=-2*pi*[31]  Gain=[31]
  M2_antiAcq_filter [65:13] : ZeroPole  Zeros=-2*pi*[65]  Poles=-2*pi*[13]  Gain=[13/65]
  M2_antiLP_filter [(1,210):(11,21)] : ZeroPole  Zeros=-2*pi*[1 210]  Poles=-2*pi*[11 21]  Gain=[1.1]
  M3_antiAcqoff_filter [82:9] : ZeroPole  Zeros=-2*pi*[82]  Poles=-2*pi*[9]  Gain=[9/82]
  M3_antiAcqon_filter [46:1.05] : ZeroPole  Zeros=-2*pi*[46]  Poles=-2*pi*[1.05]  Gain=[1.05/46]
  M3_antiLP_filter [(1,200):(10,20)] : ZeroPole  Zeros=-2*pi*[1 210]  Poles=-2*pi*[11 21]  Gain=[1.1]
  Run Acq Switch : Subsystem
  Run Acq Switch1 : Subsystem
  Out1 : Outport
  Out2 : Outport  Port=2
  Out3 : Outport  Port=3
  wires:
  Run Acq Switch1/1(Out4) -> Out3/1
  M1_white_filter [1:31]/1 -> Out1/1
  In1/1 -> M1_LP_filter [1:10]/1, LP Switch/2(In5)
  In2/1 -> M2_antiLP_filter [(1,210):(11,21)]/1, LP Switch1/2(In5)
  LP Switch2/1(Out4) -> M3_antiAcqoff_filter [82:9]/1, M3_antiAcqon_filter [46:1.05]/1
  In3/1 -> M3_antiLP_filter [(1,200):(10,20)]/1, LP Switch2/2(In5)
  LP Switch/1(Out4) -> M1_white_filter [1:31]/1
  M1_LP_filter [1:10]/1 -> LP Switch/1(In4)
  M2_antiLP_filter [(1,210):(11,21)]/1 -> LP Switch1/1(In4)
  LP Switch1/1(Out4) -> M2_antiAcq_filter [65:13]/1, Run Acq Switch/2(In5)
  M3_antiLP_filter [(1,200):(10,20)]/1 -> LP Switch2/1(In4)
  Run Acq Switch/1(Out4) -> Out2/1
  M2_antiAcq_filter [65:13]/1 -> Run Acq Switch/1(In4)
  M3_antiAcqon_filter [46:1.05]/1 -> Run Acq Switch1/1(In4)
  M3_antiAcqoff_filter [82:9]/1 -> Run Acq Switch1/2(In5)

== system IMC/MC2_control/MC2/Electronics/Coil_Driver/LP Switch ==
  In4 : Inport
  In5 : Inport  Port=2
  Switch : Switch  Threshold=0.5
  imc.sw.lp : Constant  Value=imc.sw.lp
  Out4 : Outport
  wires:
  In5/1 -> Switch/3
  In4/1 -> Switch/1
  Switch/1 -> Out4/1
  imc.sw.lp/1 -> Switch/2

== system IMC/MC2_control/MC2/Electronics/Coil_Driver/LP Switch1 ==
  In4 : Inport
  In5 : Inport  Port=2
  Switch : Switch  Threshold=0.5
  imc.sw.lp : Constant  Value=imc.sw.lp
  Out4 : Outport
  wires:
  imc.sw.lp/1 -> Switch/2
  Switch/1 -> Out4/1
  In4/1 -> Switch/1
  In5/1 -> Switch/3

== system IMC/MC2_control/MC2/Electronics/Coil_Driver/LP Switch2 ==
  In4 : Inport
  In5 : Inport  Port=2
  Switch : Switch  Threshold=0.5
  imc.sw.lp : Constant  Value=imc.sw.lp
  Out4 : Outport
  wires:
  In5/1 -> Switch/3
  In4/1 -> Switch/1
  Switch/1 -> Out4/1
  imc.sw.lp/1 -> Switch/2

== system IMC/MC2_control/MC2/Electronics/Coil_Driver/Run Acq Switch ==
  In4 : Inport
  In5 : Inport  Port=2
  Switch : Switch  Threshold=0.5
  imc.sw.runacq : Constant  Value=imc.sw.runacq
  Out4 : Outport
  wires:
  imc.sw.runacq/1 -> Switch/2
  Switch/1 -> Out4/1
  In4/1 -> Switch/1
  In5/1 -> Switch/3

== system IMC/MC2_control/MC2/Electronics/Coil_Driver/Run Acq Switch1 ==
  In4 : Inport
  In5 : Inport  Port=2
  Switch : Switch  Threshold=0.5
  imc.sw.runacq : Constant  Value=imc.sw.runacq
  Out4 : Outport
  wires:
  In5/1 -> Switch/3
  In4/1 -> Switch/1
  Switch/1 -> Out4/1
  imc.sw.runacq/1 -> Switch/2

== system IMC/MC2_control/MC2/Electronics/Coil_Output_Filters/LP Switch ==
  In4 : Inport
  In5 : Inport  Port=2
  Switch : Switch  Threshold=0.5
  imc.sw.lp : Constant  Value=imc.sw.lp
  Out4 : Outport
  wires:
  imc.sw.lp/1 -> Switch/2
  Switch/1 -> Out4/1
  In4/1 -> Switch/1
  In5/1 -> Switch/3

== system IMC/MC2_control/MC2/Electronics/Coil_Output_Filters/LP Switch1 ==
  In4 : Inport
  In5 : Inport  Port=2
  Switch : Switch  Threshold=0.5
  imc.sw.lp : Constant  Value=imc.sw.lp
  Out4 : Outport
  wires:
  In5/1 -> Switch/3
  In4/1 -> Switch/1
  Switch/1 -> Out4/1
  imc.sw.lp/1 -> Switch/2

== system IMC/MC2_control/MC2/Electronics/Coil_Output_Filters/LP Switch2 ==
  In4 : Inport
  In5 : Inport  Port=2
  Switch : Switch  Threshold=0.5
  imc.sw.lp : Constant  Value=imc.sw.lp
  Out4 : Outport
  wires:
  imc.sw.lp/1 -> Switch/2
  Switch/1 -> Out4/1
  In4/1 -> Switch/1
  In5/1 -> Switch/3

== system IMC/MC2_control/MC2/Electronics/Coil_Output_Filters/Run Acq Switch ==
  In4 : Inport
  In5 : Inport  Port=2
  Switch : Switch  Threshold=0.5
  imc.sw.runacq : Constant  Value=imc.sw.runacq
  Out4 : Outport
  wires:
  In5/1 -> Switch/3
  In4/1 -> Switch/1
  Switch/1 -> Out4/1
  imc.sw.runacq/1 -> Switch/2

== system IMC/MC2_control/MC2/Electronics/Coil_Output_Filters/Run Acq Switch1 ==
  In4 : Inport
  In5 : Inport  Port=2
  Switch : Switch  Threshold=0.5
  imc.sw.runacq : Constant  Value=imc.sw.runacq
  Out4 : Outport
  wires:
  imc.sw.runacq/1 -> Switch/2
  Switch/1 -> Out4/1
  In4/1 -> Switch/1
  In5/1 -> Switch/3
